simulink model "simple_law"  (Simulink 7.8)
settings: Solver=ode45  StartTime=0.0  StopTime=500  RelTol=1e-3
libraries: simulink x2
settings Model: Creator=Leo  LastModifiedBy=Leo

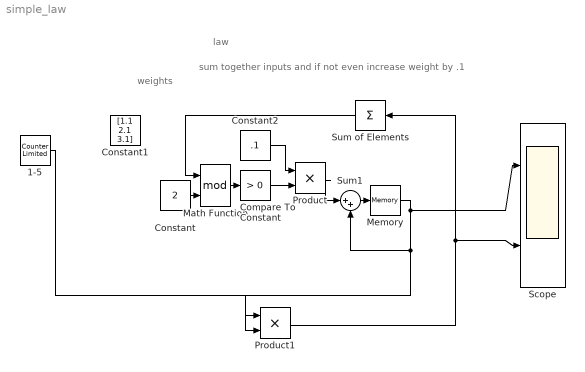
== system simple_law ==
  note: weights
  note: law
  note: sum together inputs and if not even increase weight by .1
  1-5 : simulink/Sources/Counter Limited  uplimit=5  tsamp=-1
  Compare To Constant : simulink/Logic and Bit Operations/Compare To Constant  relop=>  const=0  OutDataTypeStr=uint8
  Constant : Constant  Value=2
  Constant1 : Constant  Value=[1.1 2.1 3.1]
  Constant2 : Constant  Value=.1
  Math Function : Math  Operator=mod  SaturateOnIntegerOverflow=on
  Memory : Memory  X0=[1 3 1]
  Product : Product  RndMeth=Zero
  Product1 : Product  RndMeth=Zero
  Scope : Scope  NumInputPorts=2
      settings: YMin=-5~-5  YMax=5~5
  Sum of Elements : Sum  Inputs=+
  Sum1 : Sum  Inputs=|++
  wires:
  1-5/1 -> Product1/2
  Constant/1 -> Math Function/2
  Math Function/1 -> Compare To Constant/1
  Compare To Constant/1 -> Product/2
  Constant2/1 -> Product/1
  Product/1 -> Sum1/1
  Sum1/1 -> Memory/1
  Memory/1 -> Scope/1, Product1/1, Sum1/2
  Product1/1 -> Scope/2, Sum of Elements/1
  Sum of Elements/1 -> Math Function/1
